simulink model "non_linear_H_inf_and_compare"  (R2026a)
settings: Solver=ode15s  StartTime=0  StopTime=80  MaxStep=0.001
values from neighbouring files (symbols this model uses):
  A = [Ap                 zeros(np,nw_s)   zeros(np,nu_s) ... (first row only)    [run_hinf_suspension.m]
  Ap_c300 = mk(cmin)    [run_hinf_suspension.m]
  Ap_c8000 = mk(8000)    [run_hinf_suspension.m]
  Ap_pass = mk(c2)    [run_hinf_suspension.m]
  B1 = [Bp1; zeros(nw_s,1); zeros(nu_s,1)]    [run_hinf_suspension.m]
  Bp1 = [-1; 0; 0; 0]    [run_hinf_suspension.m]
  Bp21 = cu*Bp2*sd    [run_hinf_suspension.m]
  Bu = Bts*ones(3,1)    [run_hinf_suspension.m]
  C11 = kW*[Dws*Cp1  Cws  zeros(size(Cws,1),nu_s)]    [run_hinf_suspension.m]
  C12u = (D12'*D12)\(D12'*C12)    [run_hinf_suspension.m]
  C2 = [Cp2  zeros(size(Cp2,1),nw_s)  zeros(size(Cp2,1),nu_s)]    [run_hinf_suspension.m]
  cmax = 8000    [run_hinf_suspension.m]
  cmin = 300    [run_hinf_suspension.m]
  cu = cu*sqrt(c_target/cm)    [run_hinf_suspension.m]
  gam2 = 1.05*gam2min    [run_hinf_suspension.m]
  L = -value(R)\C2'    [run_hinf_suspension.m]
  mw1 = 0    [run_hinf_suspension.m]
  n = size(A,1)    [run_hinf_suspension.m]
  nw_s = size(Aws,1)    [run_hinf_suspension.m]
  P = value(Pv)    [run_hinf_suspension.m]
  xhat0 = zeros(n,1)    [run_hinf_suspension.m]
settings Model: Creator=ravi  LastModifiedBy=ravi

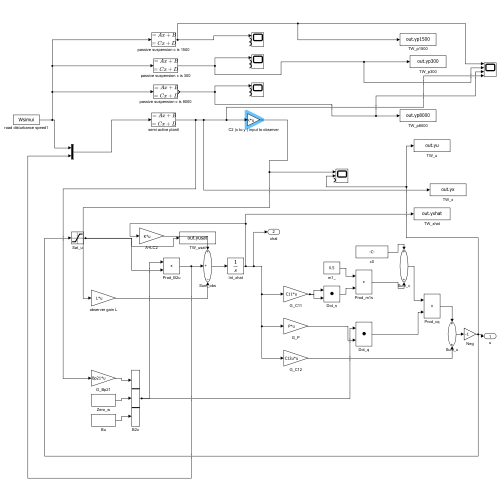
[thumbnail: Simulink's stored preview of the top-level diagram]
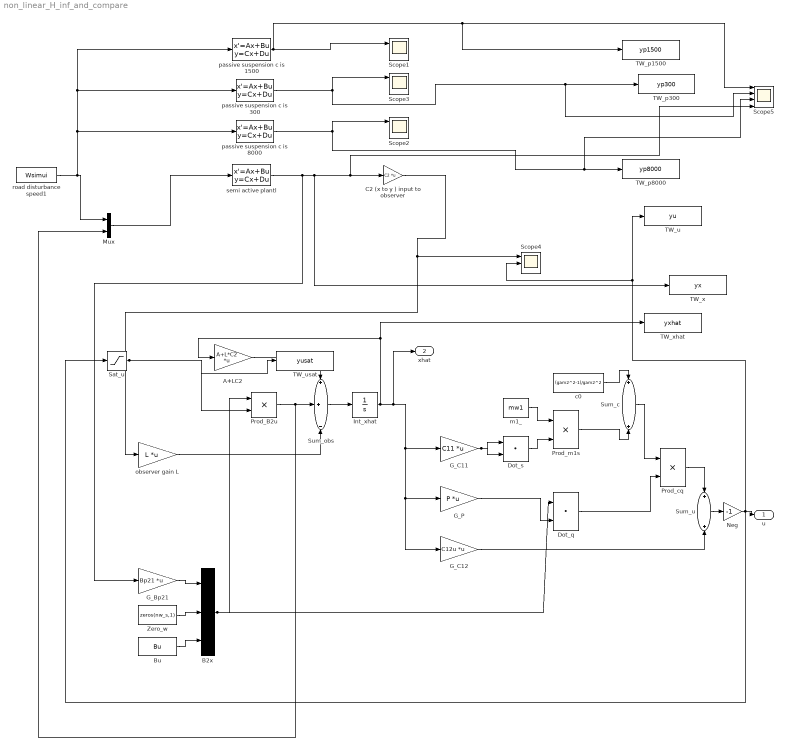
== system non_linear_H_inf_and_compare ==
  A+LC2 : Gain  Gain=A+L*C2  Multiplication=Matrix(K*u)
  B2x : Concatenate  NumInputs=3
  Bu : Constant  Value=Bu
  C2 (x to y ) input to observer : Gain  Gain=C2  Multiplication=Matrix(K*u)  SampleTime=0.001
  Dot_q : DotProduct  OutDataTypeStr=Inherit: Inherit via internal rule
  Dot_s : DotProduct  OutDataTypeStr=Inherit: Inherit via internal rule
  G_Bp21 : Gain  Gain=Bp21  Multiplication=Matrix(K*u)
  G_C11 : Gain  Gain=C11  Multiplication=Matrix(K*u)
  G_C12 : Gain  Gain=C12u  Multiplication=Matrix(K*u)
  G_P : Gain  Gain=P  Multiplication=Matrix(K*u)
  Int_xhat : Integrator  InitialCondition=xhat0
  Mux : Mux  Inputs=2
  Neg : Gain  Gain=-1
  Prod_B2u : Product
  Prod_cq : Product
  Prod_m1s : Product
  Sat_u : Saturate  UpperLimit=(cmax-cmin)/cu  LowerLimit=0  ZeroCross=off
  Scope{1..4} (4 alike) : Scope  NumInputPorts=3
      Scope1 settings: SampleTime=0.001  ActiveDisplayYMinimum=-4.4851705500318513  ActiveDisplayYMaximum=4.6046819134877417
      Scope2 settings: SampleTime=0.001  ActiveDisplayYMinimum=-4.4851705500318513  ActiveDisplayYMaximum=4.6046819134877417
      Scope3 settings: SampleTime=0.001  ActiveDisplayYMinimum=-4.4851705500318513  ActiveDisplayYMaximum=4.6046819134877417  DataLoggingVariableName=ScopeData2
      Scope4 settings: SampleTime=0.001  ActiveDisplayYMinimum=-0.17772930942849549  ActiveDisplayYMaximum=0.16151367335154929  DataLoggingVariableName=ScopeData3
  Scope5 : Scope  NumInputPorts=4
      settings: SampleTime=0.001  ActiveDisplayYMinimum=-0.22905637277424951  ActiveDisplayYMaximum=0.351364091420084  DataLoggingVariableName=ScopeData4
  Sum_c : Sum
  Sum_obs : Sum  Inputs=++-
  Sum_u : Sum
  TW_p1500 : ToWorkspace  VariableName=yp1500  SaveFormat=Timeseries  SampleTime=-1
  TW_p300 : ToWorkspace  VariableName=yp300  SaveFormat=Timeseries  SampleTime=-1
  TW_p8000 : ToWorkspace  VariableName=yp8000  SaveFormat=Timeseries  SampleTime=-1
  TW_u : ToWorkspace  VariableName=yu  SaveFormat=Timeseries  SampleTime=-1
  TW_usat : ToWorkspace  VariableName=yusat  SaveFormat=Timeseries  SampleTime=-1
  TW_x : ToWorkspace  VariableName=yx  SaveFormat=Timeseries  SampleTime=-1
  TW_xhat : ToWorkspace  VariableName=yxhat  SaveFormat=Timeseries  SampleTime=-1
  Zero_w : Constant  Value=zeros(nw_s,1)
  c0 : Constant  Value=(gam2^2-1)/gam2^2
  m1_ : Constant  Value=mw1
  observer gain L : Gain  Gain=L  Multiplication=Matrix(K*u)
  passive suspension c is 1500 : StateSpace  A=Ap_pass  B=Bp1  C=eye(4)  D=zeros(4,1)  InitialCondition=0
  passive suspension c is 300 : StateSpace  A=Ap_c300  B=Bp1  C=eye(4)  D=zeros(4,1)  InitialCondition=0
  passive suspension c is 8000 : StateSpace  A=Ap_c8000  B=Bp1  C=eye(4)  D=zeros(4,1)  InitialCondition=0
  road disturbance speed1 : FromWorkspace  VariableName=Wsimui  OutDataTypeStr=double  SampleTime=0.001
  semi active plantl : StateSpace  A=A  B=[B1 eye(n)]  C=eye(n)  D=zeros(n,1+n)  InitialCondition=0  ParameterTunability=Unconstrained  ContinuousStateAttributes='original'
  u : Outport
  xhat : Outport  Port=2
  wires:
  A+LC2/1 -> Sum_obs/1
  B2x/1 -> Prod_B2u/1, Dot_q/1
  Prod_B2u/1 -> Sum_obs/2, Mux/2
  observer gain L/1 -> Sum_obs/3
  Sum_obs/1 -> Int_xhat/1
  G_Bp21/1 -> B2x/1
  Zero_w/1 -> B2x/2
  Bu/1 -> B2x/3
  G_C11/1 -> Dot_s/1, Dot_s/2
  m1_/1 -> Prod_m1s/1
  Dot_s/1 -> Prod_m1s/2
  c0/1 -> Sum_c/1
  Prod_m1s/1 -> Sum_c/2
  G_P/1 -> Dot_q/2
  Sum_c/1 -> Prod_cq/1
  Dot_q/1 -> Prod_cq/2
  Prod_cq/1 -> Sum_u/1
  G_C12/1 -> Sum_u/2
  Sum_u/1 -> Neg/1
  C2 (x to y ) input to observer/1 -> Scope4/1, observer gain L/1
  Neg/1 -> TW_u/1, Scope4/2, Sat_u/1, u/1
  Mux/1 -> semi active plantl/1
  road disturbance speed1/1 -> passive suspension c is 8000/1, passive suspension c is 300/1, passive suspension c is 1500/1, Mux/1
  passive suspension c is 1500/1 -> Scope1/1, Scope5/1, TW_p1500/1
  passive suspension c is 300/1 -> Scope3/1, Scope5/2, TW_p300/1
  passive suspension c is 8000/1 -> Scope2/1, Scope5/3, TW_p8000/1
  Sat_u/1 -> Prod_B2u/2, TW_usat/1
  Int_xhat/1 -> TW_xhat/1, A+LC2/1, G_P/1, G_C12/1, G_C11/1, xhat/1
  semi active plantl/1 -> G_Bp21/1, Scope5/4, C2 (x to y ) input to observer/1, TW_x/1
